simulink library "energyStorageDevices"  (R2013a)
settings: Solver=ode3  StartTime=0.0  StopTime=10.0  RelTol=1e-3
undefined symbols (not defined in the file): battery, nr
libraries: goto x5
settings Model: Creator=torstebo  LastModifiedBy=Michel

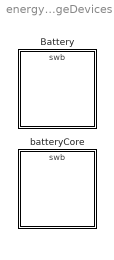
== system energyStorageDevices ==
  Battery : Subsystem  Tag=EmergencyBattery  mask{swbId=1, battery=battery(1)}
  batteryCore : Subsystem  Tag=EmergencyBattery  mask{swbId=1, battery=battery(1)}

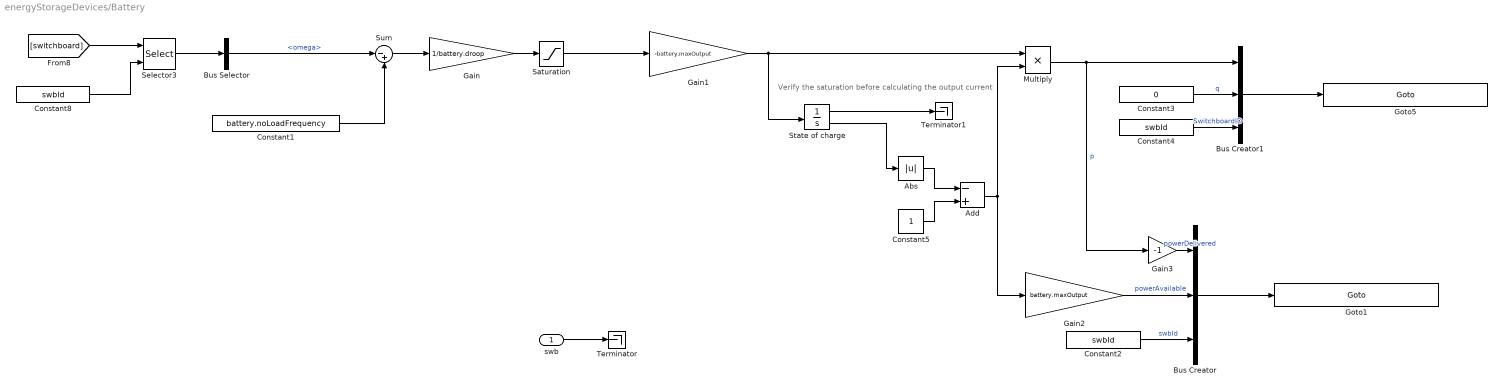
== system energyStorageDevices/Battery ==
  note: Verify the saturation before calculating the output current
  swb : Inport
  Abs : Abs
  Add : Sum  Inputs=-+
  Bus Creator : BusCreator  Inputs=3  OutDataTypeStr=Bus: EmergencyBattery  NonVirtualBus=on
  Bus Selector : BusSelector  OutputSignals=omega
  Bus Creator1 : BusCreator  Inputs='p','q','SwitchboardID'  OutDataTypeStr=Bus: powerLoadsBus  NonVirtualBus=on
  Constant1 : Constant  Value=battery.noLoadFrequency  OutDataTypeStr=Inherit: Inherit via back propagation
  Constant2 : Constant  Value=swbId  OutDataTypeStr=Inherit: Inherit via back propagation
  Constant3 : Constant  Value=0  OutDataTypeStr=Inherit: Inherit via back propagation
  Constant4 : Constant  Value=swbId  OutDataTypeStr=Inherit: Inherit via back propagation
  Constant5 : Constant
  Constant8 : Constant  Value=swbId  OutDataTypeStr=Inherit: Inherit via back propagation
  Gain : Gain  Gain=1/battery.droop
  Gain1 : Gain  Gain=-battery.maxOutput
  Gain2 : Gain  Gain=battery.maxOutput  ParamDataTypeStr=double  OutDataTypeStr=double
  Gain3 : Gain  Gain=-1
  Goto1 : goto/Goto  GotoTag=sprintf('EmergencyBattery%d',swbId)
  Goto5 : goto/Goto  GotoTag=sprintf('PowerEmergencyBatteries%d',swbId)
  Multiply : Product  Inputs=**
  Saturation : Saturate  UpperLimit=1  LowerLimit=0
  Selector3 : Selector  IndexOptions=Index vector (port)  Indices=[nr]  OutputSizes=1
  State of charge : Integrator  InitialCondition=battery.initialCapacity  LimitOutput=on  UpperSaturationLimit=battery.maxCapacity  LowerSaturationLimit=0  ShowSaturationPort=on
  Sum : Sum  Inputs=|-+
  Terminator : Terminator
  Terminator1 : Terminator
  wires:
  swb/1 -> Terminator/1
  Bus Selector/1 -> Sum/1  "<omega>"
  [switchboard] -> Selector3/1
  Constant8/1 -> Selector3/2
  Selector3/1 -> Bus Selector/1
  Constant1/1 -> Sum/2
  Sum/1 -> Gain/1
  Gain/1 -> Saturation/1
  Saturation/1 -> Gain1/1
  Gain2/1 -> Bus Creator/2  "powerAvailable"
  Bus Creator/1 -> Goto1/1
  Bus Creator1/1 -> Goto5/1
  Constant3/1 -> Bus Creator1/2  "q"
  Constant4/1 -> Bus Creator1/3  "SwitchboardID"
  Constant2/1 -> Bus Creator/3  "swbId"
  Gain3/1 -> Bus Creator/1  "powerDelivered"
  Multiply/1 -> Gain3/1, Bus Creator1/1  "p"
  Add/1 -> Gain2/1, Multiply/2
  Abs/1 -> Add/1
  Constant5/1 -> Add/2
  State of charge/2 -> Abs/1
  Gain1/1 -> Multiply/1, State of charge/1
  State of charge/1 -> Terminator1/1

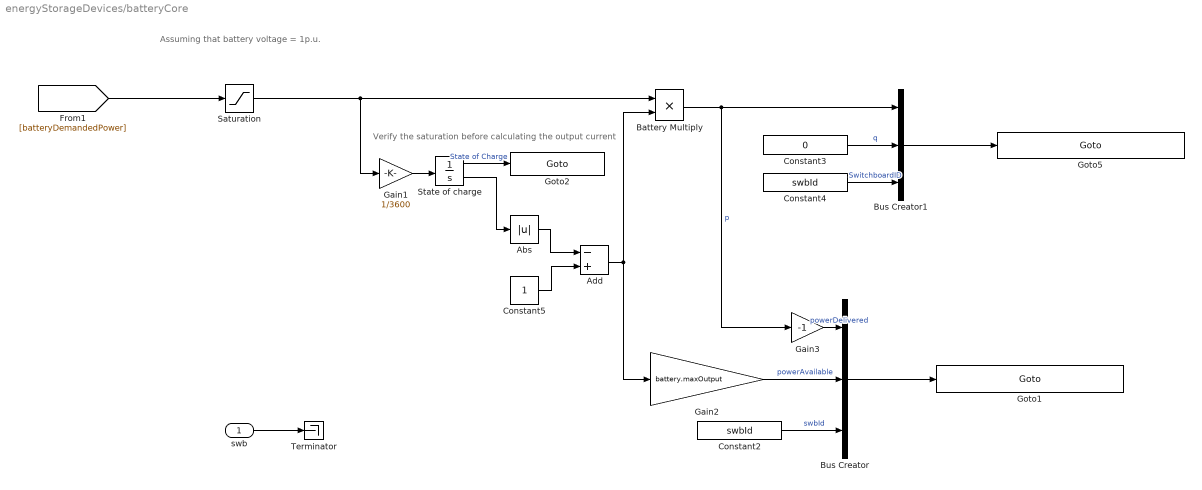
== system energyStorageDevices/batteryCore ==
  note: Assuming that battery voltage = 1p.u.
  note: Verify the saturation before calculating the output current
  swb : Inport
  Abs : Abs
  Add : Sum  Inputs=-+
  Battery Multiply : Product  Inputs=**
  Bus Creator : BusCreator  Inputs=3  OutDataTypeStr=Bus: EmergencyBattery  NonVirtualBus=on
  Bus Creator1 : BusCreator  Inputs='p','q','SwitchboardID'  OutDataTypeStr=Bus: powerLoadsBus  NonVirtualBus=on
  Constant2 : Constant  Value=swbId  OutDataTypeStr=Inherit: Inherit via back propagation
  Constant3 : Constant  Value=0  OutDataTypeStr=Inherit: Inherit via back propagation
  Constant4 : Constant  Value=swbId  OutDataTypeStr=Inherit: Inherit via back propagation
  Constant5 : Constant
  Gain1 : Gain  Gain=1/3600
  Gain2 : Gain  Gain=battery.maxOutput  ParamDataTypeStr=double  OutDataTypeStr=double
  Gain3 : Gain  Gain=-1
  Goto1 : goto/Goto  GotoTag=sprintf('EmergencyBattery%d',swbId)
  Goto2 : goto/Goto  GotoTag=sprintf('batterySOC%d',swbId)
  Goto5 : goto/Goto  GotoTag=sprintf('PowerEmergencyBatteries%d',swbId)
  Saturation : Saturate  UpperLimit=battery.maxOutput * battery.maxCapacity  LowerLimit=-battery.maxInput * battery.maxCapacity
  State of charge : Integrator  InitialCondition=battery.initialCharge * battery.maxCapacity  LimitOutput=on  UpperSaturationLimit=battery.maxCapacity  LowerSaturationLimit=0  ShowSaturationPort=on
  Terminator : Terminator
  wires:
  swb/1 -> Terminator/1
  Bus Creator1/1 -> Goto5/1
  Constant3/1 -> Bus Creator1/2  "q"
  Constant4/1 -> Bus Creator1/3  "SwitchboardID"
  Add/1 -> Gain2/1, Battery Multiply/2
  Abs/1 -> Add/1
  Constant5/1 -> Add/2
  State of charge/2 -> Abs/1
  Saturation/1 -> Battery Multiply/1, Gain1/1
  State of charge/1 -> Goto2/1  "State of Charge"
  [batteryDemandedPower] -> Saturation/1
  Gain1/1 -> State of charge/1
  Gain2/1 -> Bus Creator/2  "powerAvailable"
  Bus Creator/1 -> Goto1/1
  Constant2/1 -> Bus Creator/3  "swbId"
  Gain3/1 -> Bus Creator/1  "powerDelivered"
  Battery Multiply/1 -> Gain3/1, Bus Creator1/1  "p"
